simulink model "compare_psk"  (Simulink 7.2)
settings: Solver=ode45  StartTime=0.0  StopTime=inf  RelTol=1e-3
values from neighbouring files (symbols this model uses):
  const = inphase + quadr*j    [compare_PSK_mod.m]    (also in signal.m)
  EbNodB = EbNoVec(n)    [compare_PSK_mod.m]
libraries: commdigbbndam3 x2, commchan3 x1, commsink2 x1, commrandsrc2 x1
settings Model: Creator=nazarova_a_a  LastModifiedBy=Svetlana
settings DataIOCC: LimitDataPoints=off  SaveOutput=off  SaveTime=off  SignalLoggingName=sigsOut
settings OptimizationCC: BlockReduction=off  BooleanDataType=off  InitFltsAndDblsToZero=on
settings DebuggingCC: SaveWithParameterizedLinksMsg=none  SignalResolutionControl=TryResolveAllWithWarning  SolverPrmCheckMsg=none  MultiTaskDSMMsg=warning  MultiTaskCondExecSysMsg=none  StrictBusMsg=None
settings HardwareCC: TargetUnknown=on
settings RTWCC: IncludeERTFirstTime=on
settings GRTTargetCC: TargetFcnLib=ansi_tfl_tmw.mat

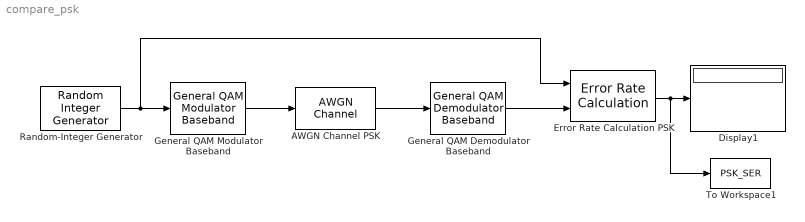
== system compare_psk ==
  AWGN Channel PSK : commchan3/AWGN Channel  SystemSampleTime=-1  seed=1237  noiseMode="Signal to noise ratio  (Es/No)"  EbNodB=10  EsNodB=EbNodB+10*log10(4)  SNRdB=10  bitsPerSym=1  Ps=sum((abs(const)).^2)/length(const)  Tsym=1  variance=1
  Display1 : Display
  Error Rate Calculation PSK : commsink2/Error Rate Calculation  N=0  st_delay=0  cp_mode=Entire frame  subframe=[]  PMode=Port  WsName=ErrorVec  RsMode2=off  stop=on  numErr=1e4  maxBits=steps
  General QAM Demodulator Baseband : commdigbbndam3/General QAM Demodulator Baseband  DialogController=commDDGCreate  DialogControllerArgs=DataTag0  SigCon=const  OutType=Integer  DecType=Hard decision  VarSource=Dialog  Variance=1  outDtypeBit=Inherit via internal rule  outDtype=Inherit via internal rule  roundingMode=Floor  overflowMode=Wrap  sigConstWordLen=16  accum1WordLen=32  accum1FracLen=30  prodInWordLen=32  prodInFracLen=30  prodOutWordLen=32  prodOutFracLen=30  accum2WordLen=32  accum2FracLen=30  accum3WordLen=32  accum3FracLen=30  nsiWordLen=32  nsiFracLen=30  invn0WordLen=16  invn0FracLen=8  outputWordLen=32  outputFracLen=30
  General QAM Modulator Baseband : commdigbbndam3/General QAM Modulator Baseband  DialogController=commDDGCreate  DialogControllerArgs=DataTag1  SigCon=const  outDtype=double  outWordLen=16  outUDDataType=sfix(16)  outFracLenMode=Best precision  outFracLen=15
  Random-Integer Generator : commrandsrc2/Random Integer Generator  SystemSampleTime=-1  mul=length(const)  seed=12345  Ts=1  frameBased=on  sampPerFrame=10000  orient=off  outDataType=double
  To Workspace1 : ToWorkspace  VariableName=PSK_SER  SampleTime=-1  SaveFormat=Array
      settings: MaxDataPoints=1
  wires:
  AWGN Channel PSK/1 -> General QAM Demodulator Baseband/1
  General QAM Demodulator Baseband/1 -> Error Rate Calculation PSK/2
  Error Rate Calculation PSK/1 -> Display1/1, To Workspace1/1
  General QAM Modulator Baseband/1 -> AWGN Channel PSK/1
  Random-Integer Generator/1 -> Error Rate Calculation PSK/1, General QAM Modulator Baseband/1
